simulink model "P2SerialReceiveb"  (R2020b)
settings: Solver=VariableStepAuto  StartTime=0.0  StopTime=inf  RelTol=1e-3
model workspace (MAT data in the model file):
  dt = Simulink.Parameter
  dt.Value = 0.01
  dt.DataType = 'auto'
  dt.Dimensions = [1 1]
undefined symbols (not defined in the file or in its folder): serial
libraries: instrumentlib x2
settings Model: EnablePacing=on  Creator=eber_  LastModifiedBy=eber_

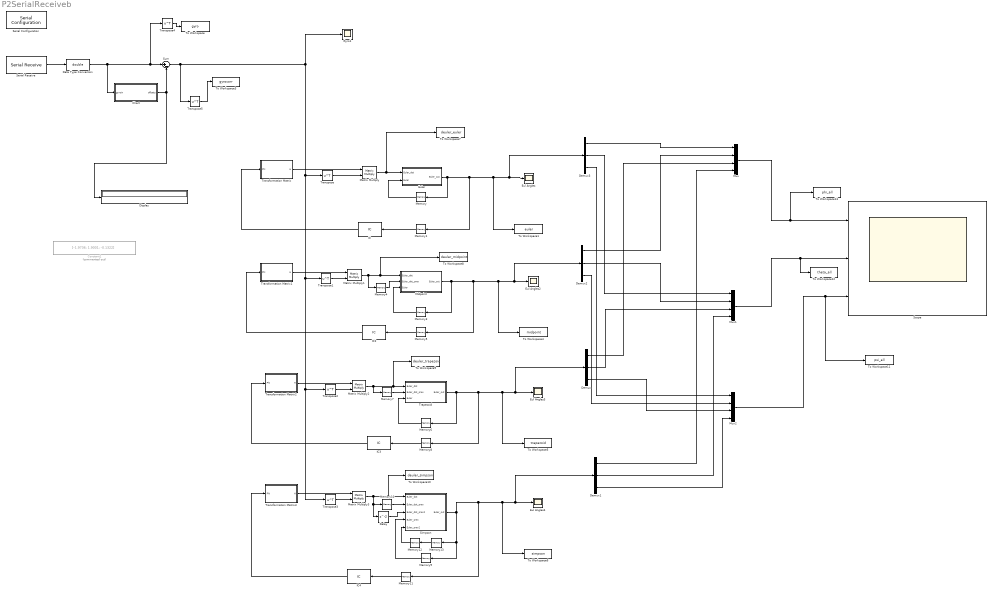
== system P2SerialReceiveb ==
  Chart : Stateflow chart  TreatAsAtomicUnit=on
  Constant1 : Constant  Commented=on  Value=[-1.9736; 1.9001; -0.1322]
  Data Type Conversion : DataTypeConversion  OutDataTypeStr=double
  Delay : Delay
  Demux{,1..3} (4 alike) : Demux  Outputs=3
  Display : Display
  Eul Angles{,2..4} (4 alike) : Scope
  Euler : MATLAB Function  TreatAsAtomicUnit=on
  Gyro1 : Scope
  IC{,2..4} (4 alike) : InitialCondition  Value=[0; 0; 0]
  Matrix Multiply{,1..3} (4 alike) : Product  Multiplication=Matrix(*)
  Memory{,1,3..8,10..11} (10 alike) : Memory
  Memory12 : Memory  InheritSampleTime=on
  Memory13 : Memory  InheritSampleTime=on
  Memory9 : Memory  InheritSampleTime=on
  Midpoint : MATLAB Function  TreatAsAtomicUnit=on
  Mux : Mux
  Mux1 : Mux
  Mux2 : Mux
  Scope : Scope  NumInputPorts=3
  Serial Configuration : instrumentlib/Serial Configuration  Priority=-200000  ComPortMenu=<Please select a port...>  ComPort=COM3  ObjConstructor=serial('COM3');  BaudRate=115200  DataBits=8  Parity=none  StopBits=1  FlowControl=none  Timeout=10  ByteOrder=LittleEndian
  Serial Receive : instrumentlib/Serial Receive  ComPortMenu=<Please select a port...>  ComPort=COM3  ObjConstructor=serial('COM3');  Terminator=<none>  DataSize="[1  3]"  DataType=single  EnableBlockingMode=on  ActionDataUnavailable=Output last received value  CustomValue=0  SampleTime=0.02
  Simpson : MATLAB Function  TreatAsAtomicUnit=on
  Sum : Sum  Inputs=|+-
  To Workspace : ToWorkspace  VariableName=gyro  SaveFormat=Structure With Time  SampleTime=-1
  To Workspace1 : ToWorkspace  VariableName=euler  SaveFormat=Structure With Time  SampleTime=-1
  To Workspace10 : ToWorkspace  VariableName=deuler_simpson  SaveFormat=Structure With Time  SampleTime=-1
  To Workspace11 : ToWorkspace  VariableName=psi_all  SaveFormat=Structure With Time  SampleTime=-1
  To Workspace12 : ToWorkspace  VariableName=theta_all  SaveFormat=Structure With Time  SampleTime=-1
  To Workspace13 : ToWorkspace  VariableName=phi_all  SaveFormat=Structure With Time  SampleTime=-1
  To Workspace3 : ToWorkspace  VariableName=gyrocorr  SaveFormat=Structure With Time  SampleTime=-1
  To Workspace4 : ToWorkspace  VariableName=midpoint  SaveFormat=Structure With Time  SampleTime=-1
  To Workspace5 : ToWorkspace  VariableName=trapezoid  SaveFormat=Structure With Time  SampleTime=-1
  To Workspace6 : ToWorkspace  VariableName=simpson  SaveFormat=Structure With Time  SampleTime=-1
  To Workspace7 : ToWorkspace  VariableName=deuler_euler  SaveFormat=Structure With Time  SampleTime=-1
  To Workspace8 : ToWorkspace  VariableName=deuler_midpoint  SaveFormat=Structure With Time  SampleTime=-1
  To Workspace9 : ToWorkspace  VariableName=deuler_trapezoid  SaveFormat=Structure With Time  SampleTime=-1
  Transformation Matrix : MATLAB Function  TreatAsAtomicUnit=on
  Transformation Matrix1 : MATLAB Function  TreatAsAtomicUnit=on
  Transformation Matrix2 : MATLAB Function  TreatAsAtomicUnit=on
  Transformation Matrix3 : MATLAB Function  TreatAsAtomicUnit=on
  Transpose{,1..5} (6 alike) : Math  Operator=transpose  SaturateOnIntegerOverflow=on
  Trapezoid : MATLAB Function  TreatAsAtomicUnit=on
  wires:
  Serial Receive/1 -> Data Type Conversion/1
  Data Type Conversion/1 -> Transpose4/1, Sum/1, Chart/1(gyroIn)
  Chart/1(offsets) -> Sum/2, Display/1
  Euler/1(Euler_out) -> Memory/1, Memory1/1, To Workspace1/1, Eul Angles/1, Demux3/1
  IC/1 -> Transformation Matrix/1(Phi)
  Memory1/1 -> IC/1
  Memory/1 -> Euler/2(Euler)
  Transformation Matrix/1(H) -> Matrix Multiply/1
  Transpose/1 -> Matrix Multiply/2
  Matrix Multiply/1 -> To Workspace7/1, Euler/1(Euler_dot)
  Matrix Multiply1/1 -> Memory4/1, To Workspace8/1, Midpoint/1(Euler_dot)
  Transpose1/1 -> Matrix Multiply1/2
  Transformation Matrix1/1(H) -> Matrix Multiply1/1
  Memory3/1 -> Midpoint/3(Euler)
  Memory5/1 -> IC2/1
  IC2/1 -> Transformation Matrix1/1(Phi)
  Midpoint/1(Euler_out) -> Demux2/1, Eul Angles2/1, To Workspace4/1, Memory5/1, Memory3/1
  Memory4/1 -> Midpoint/2(Euler_dot_prev)
  Memory7/1 -> Trapezoid/2(Euler_dot_prev)
  Trapezoid/1(Euler_out) -> Memory6/1, Memory8/1, To Workspace5/1, Demux/1, Eul Angles3/1
  IC3/1 -> Transformation Matrix2/1(Phi)
  Memory8/1 -> IC3/1
  Memory6/1 -> Trapezoid/3(Euler)
  Transformation Matrix2/1(H) -> Matrix Multiply2/1
  Transpose2/1 -> Matrix Multiply2/2
  Matrix Multiply2/1 -> To Workspace9/1, Trapezoid/1(Euler_dot), Memory7/1
  Matrix Multiply3/1 -> Delay/1, Memory10/1, To Workspace10/1, Simpson/1(Euler_dot)
  Sum/1 -> Transpose5/1, Transpose1/1, Transpose3/1, Transpose2/1, Transpose/1, Gyro1/1
  Transpose3/1 -> Matrix Multiply3/2
  Transformation Matrix3/1(H) -> Matrix Multiply3/1
  Memory9/1 -> Simpson/4(Euler_prev)
  Memory11/1 -> IC4/1
  IC4/1 -> Transformation Matrix3/1(Phi)
  Simpson/1(Euler_out) -> Memory9/1, Memory13/1, Demux1/1, Eul Angles4/1, To Workspace6/1, Memory11/1
  Memory10/1 -> Simpson/2(Euler_dot_prev)
  Memory12/1 -> Simpson/5(Euler_prev2)
  Delay/1 -> Simpson/3(Euler_dot_prev2)
  Demux3/1 -> Mux/1
  Demux2/1 -> Mux/2
  Demux/1 -> Mux/3
  Demux1/1 -> Mux/4
  Demux3/2 -> Mux1/1
  Demux2/2 -> Mux1/2
  Demux/2 -> Mux1/3
  Demux1/2 -> Mux1/4
  Demux3/3 -> Mux2/1
  Demux2/3 -> Mux2/2
  Demux/3 -> Mux2/3
  Demux1/3 -> Mux2/4
  Mux/1 -> To Workspace13/1, Scope/1
  Mux1/1 -> To Workspace12/1, Scope/2
  Mux2/1 -> To Workspace11/1, Scope/3
  Memory13/1 -> Memory12/1
  Transpose4/1 -> To Workspace/1
  Transpose5/1 -> To Workspace3/1

== matlab function P2SerialReceiveb/Euler ==
  data: Euler_dot input; Euler_out output; Euler input
function Euler_out = fcn(Euler_dot, Euler)
dt = 0.0125;
phi_dot = Euler_dot(1);
theta_dot = Euler_dot(2);
psi_dot = Euler_dot(3);

phi = Euler(1);
theta = Euler(2);
psi = Euler(3);


phi = phi + dt*phi_dot;
theta = theta + dt*theta_dot;
psi = psi + dt*psi_dot;

Euler_out = [phi; theta; psi];

== matlab function P2SerialReceiveb/Transformation Matrix ==
  data: Phi input; H output
function H = fcn(Phi)
Phi = deg2rad(Phi);

phi = Phi(1);
theta = Phi(2);
psi = Phi(3);

H = [1 tan(theta)*sin(phi) tan(theta)*cos(phi);
    0 cos(phi) -sin(phi);
    0 sin(phi)/cos(theta) cos(phi)/cos(theta)];

== matlab function P2SerialReceiveb/Midpoint ==
  data: Euler_dot input; Euler_dot_prev input; Euler_out output; Euler input
function Euler_out = fcn(Euler_dot, Euler_dot_prev, Euler)
dt = 0.0125;

phi_dot = Euler_dot(1);
theta_dot = Euler_dot(2);
psi_dot = Euler_dot(3);


phi_dot_prev = Euler_dot_prev(1);
theta_dot_prev = Euler_dot_prev(2);
psi_dot_prev = Euler_dot_prev(3);


phi = Euler(1);
theta = Euler(2);
psi = Euler(3);


phi = phi + dt*((phi_dot + phi_dot_prev)/2);
theta = theta + dt*((theta_dot + theta_dot_prev)/2);
psi = psi + dt*((psi_dot + psi_dot_prev)/2);

Euler_out = [phi; theta; psi];

== matlab function P2SerialReceiveb/Transformation Matrix1 ==
  data: Phi input; H output
function H = fcn(Phi)
Phi = deg2rad(Phi);

phi = Phi(1);
theta = Phi(2);
psi = Phi(3);

H = [1 tan(theta)*sin(phi) tan(theta)*cos(phi);
    0 cos(phi) -sin(phi);
    0 sin(phi)/cos(theta) cos(phi)/cos(theta)];

== stateflow chart P2SerialReceiveb/Chart ==
  state dataAcquisition
    entry:
    offsets = [-2.042; 1.889; -0.02741];
    %offsets = [0.001564; -0.001017; 0.01126];
    phiSum = 0;
    thetaSum = 0;
    psiSum = 0;
    counter = 0;
    during:
    phi = gyroIn(1);
    theta = gyroIn(2);
    psi = gyroIn(3);
    counter = counter + 1;
    phiSum = phiSum + phi;
    thetaSum = thetaSum + theta;
    psiSum = psiSum + psi;
  state average
    entry:
    phiOffset = phiSum/counter;
    thetaOffset = thetaSum/counter;
    psiOffset = psiSum/counter;
    during:
    offsets = [phiOffset; thetaOffset; psiOffset];
  (default) -> dataAcquisition
  dataAcquisition -> average : after(10, sec)
  data: gyroIn input; offsets output; counter local; phi local; phiOffset local; phiSum local; psi local; psiOffset local; psiSum local; theta local; thetaOffset local; thetaSum local

== matlab function P2SerialReceiveb/Trapezoid ==
  data: Euler_dot input; Euler_dot_prev input; Euler_out output; Euler input
function Euler_out = fcn(Euler_dot, Euler_dot_prev, Euler)
dt = 0.0125;

phi_dot = Euler_dot(1);
theta_dot = Euler_dot(2);
psi_dot = Euler_dot(3);


phi_dot_prev = Euler_dot_prev(1);
theta_dot_prev = Euler_dot_prev(2);
psi_dot_prev = Euler_dot_prev(3);


phi = Euler(1);
theta = Euler(2);
psi = Euler(3);


phi = phi + dt*phi_dot - dt*((phi_dot - phi_dot_prev)/2);
theta = theta + dt*theta_dot - dt*((theta_dot - theta_dot_prev)/2);
psi = psi + dt*psi_dot - dt*((psi_dot - psi_dot_prev)/2);

Euler_out = [phi; theta; psi];

== matlab function P2SerialReceiveb/Transformation Matrix2 ==
  data: Phi input; H output
function H = fcn(Phi)
Phi = deg2rad(Phi);

phi = Phi(1);
theta = Phi(2);
psi = Phi(3);

H = [1 tan(theta)*sin(phi) tan(theta)*cos(phi);
    0 cos(phi) -sin(phi);
    0 sin(phi)/cos(theta) cos(phi)/cos(theta)];

== matlab function P2SerialReceiveb/Transformation Matrix3 ==
  data: Phi input; H output
function H = fcn(Phi)
Phi = deg2rad(Phi);

phi = Phi(1);
theta = Phi(2);
psi = Phi(3);

H = [1 tan(theta)*sin(phi) tan(theta)*cos(phi);
    0 cos(phi) -sin(phi);
    0 sin(phi)/cos(theta) cos(phi)/cos(theta)];

== matlab function P2SerialReceiveb/Simpson ==
  data: Euler_dot input; Euler_dot_prev input; Euler_dot_prev2 input; Euler_out output; Euler_prev input; Euler_prev2 input
function Euler_out = fcn(Euler_dot, Euler_dot_prev, Euler_dot_prev2, Euler_prev, Euler_prev2)
dt = 0.0125;

phi_dot = Euler_dot(1);
theta_dot = Euler_dot(2);
psi_dot = Euler_dot(3);

phi_dot_prev = Euler_dot_prev(1);
theta_dot_prev = Euler_dot_prev(2);
psi_dot_prev = Euler_dot_prev(3);

phi_dot_prev2 = Euler_dot_prev2(1);
theta_dot_prev2 = Euler_dot_prev2(2);
psi_dot_prev2 = Euler_dot_prev2(3);

phi_prev = Euler_prev(1);
theta_prev = Euler_prev(2);
psi_prev = Euler_prev(3);

phi_prev2 = Euler_prev2(1);
theta_prev2 = Euler_prev2(2);
psi_prev2 = Euler_prev2(3);

phi = phi_prev2 + (dt/3)*(phi_dot_prev2 + 4*phi_dot_prev + phi_dot);
theta = theta_prev2 + (dt/3)*(theta_dot_prev2 + 4*theta_dot_prev + theta_dot);
psi = psi_prev2 + (dt/3)*(psi_dot_prev2 + 4*psi_dot_prev + psi_dot);

Euler_out = [phi; theta; psi];
